simulink model "duSystem"  (Simulink 7.5)
settings: Solver=ode45  StartTime=0.0  StopTime=3  RelTol=1e-3
settings Model: Creator=Dranik_win  LastModifiedBy=Dranik_win

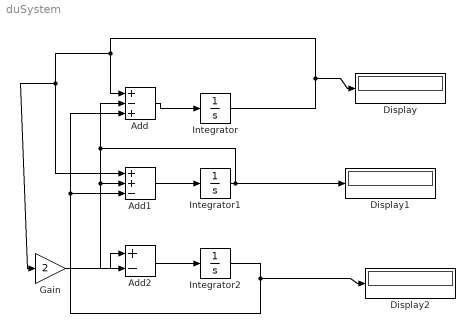
== system duSystem ==
  Add : Sum  Inputs=+-+  OutDataType=fixdt(1, 16)  OutScaling=2^-10
  Add1 : Sum  Inputs=++-  OutDataType=fixdt(1, 16)  OutScaling=2^-10
  Add2 : Sum  Inputs=+-  OutDataType=fixdt(1, 16)  OutScaling=2^-10
  Display : Display
  Display1 : Display
  Display2 : Display
  Gain : Gain  Gain=2  ParameterDataType=fixdt(1, 16)  ParameterScaling=2^0  OutDataType=fixdt(1, 16)  OutScaling=2^0
  Integrator : Integrator  InitialCondition=1
  Integrator1 : Integrator  InitialCondition=1
  Integrator2 : Integrator  InitialCondition=1
  wires:
  Integrator/1 -> Add/1, Add1/1, Gain/1, Display/1
  Add/1 -> Integrator/1
  Add1/1 -> Integrator1/1
  Add2/1 -> Integrator2/1
  Integrator1/1 -> Add/2, Add1/2, Add2/2, Display1/1
  Integrator2/1 -> Add/3, Add1/3, Display2/1
  Gain/1 -> Add2/1
